simulink model "SensorlessBDC"  (R2025a)
settings: Solver=FixedStepDiscrete  StartTime=0.0  StopTime=1  RelTol=1e-3  EnableMultiTasking=on
undefined symbols (not defined in the file or in its folder): A, B, observer_params, pi_params, robot_params, tf_den, tf_num, Ts
libraries: simulink x4, mcbhdlcontrolslib x2, SignalEditorBlockLib x1
settings Model: Creator=Evan Wu  LastModifiedBy=Evan Wu
settings SolverCC: AutoInsertRateTranBlk=on
settings DataIOCC: SaveOutput=off  SaveTime=off
settings OptimizationCC: DefaultParameterBehavior=Inlined  InlineInvariantSignals=on  EnhancedBackFolding=on  PassReuseOutputArgsAs=Individual arguments  StateBitsets=on  DataBitsets=on  ZeroExternalMemoryAtStartup=off  ZeroInternalMemoryAtStartup=off  NoFixptDivByZeroProtection=on  LifeSpan=1  OptimizeBlockOrder=speed  DifferentSizesBufferReuse=on  EfficientTunableParamExpr=on
settings DebuggingCC: AlgebraicLoopMsg=error  ParameterTunabilityLossMsg=error
settings HardwareCC: ProdBitPerPointer=32.0  ProdBitPerSizeT=32.0  ProdBitPerPtrDiffT=32.0  ProdLargestAtomicFloat=None  ProdIntDivRoundTo=Floor  ProdWordSize=32.0  ProdHWDeviceType=Generic->Custom
settings SFSimCC: MATLABDynamicMemAlloc=off
settings RTWCC: SystemTargetFile=ert.tlc  TLCOptions=-p0  GenCodeOnly=on  TemplateMakefile=ert_default_tmf  GenerateReport=on  RTWVerbose=off  IncludeHyperlinkInReport=on  LaunchReport=on  Description=Embedded Coder
settings CodeAppCC: ForceParamTrailComments=on  IgnoreCustomStorageClasses=off  OperatorAnnotations=on  SimulinkDataObjDesc=on  SFDataObjDesc=on  CustomSymbolStrGlobalVar=rt$N$M  CustomSymbolStrType=$N$M  CustomSymbolStrFcn=$N$M$F  CustomSymbolStrMacro=$N$M  InsertBlockDesc=on
settings ERTTargetCC: ExtModeTransport=0.0  ExtModeStaticAlloc=off  ExtModeMexFile=ext_comm  ExtModeIntrfLevel=Level1  RootIOFormat=Structure reference  ERTCustomFileTemplate=example_file_process.tlc  TargetLangStandard=C99 (ISO)  CodeReplacementLibrary=ISO_C  GenerateSampleERTMain=on  IncludeMdlTerminateFcn=off  SuppressErrorStatus=on  SupportAbsoluteTime=off  PurelyIntegerCode=on  SupportNonFinite=off  SupportComplex=off

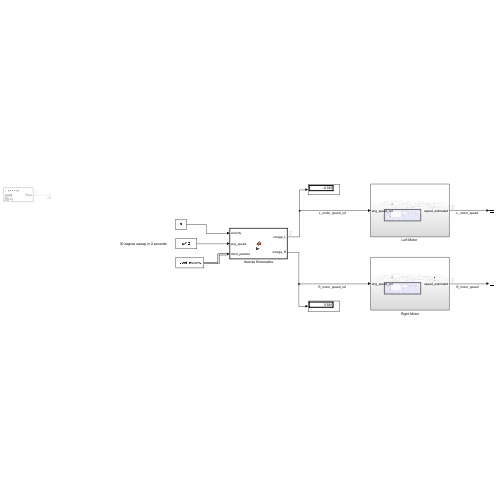
[thumbnail: Simulink's stored preview of the top-level diagram]
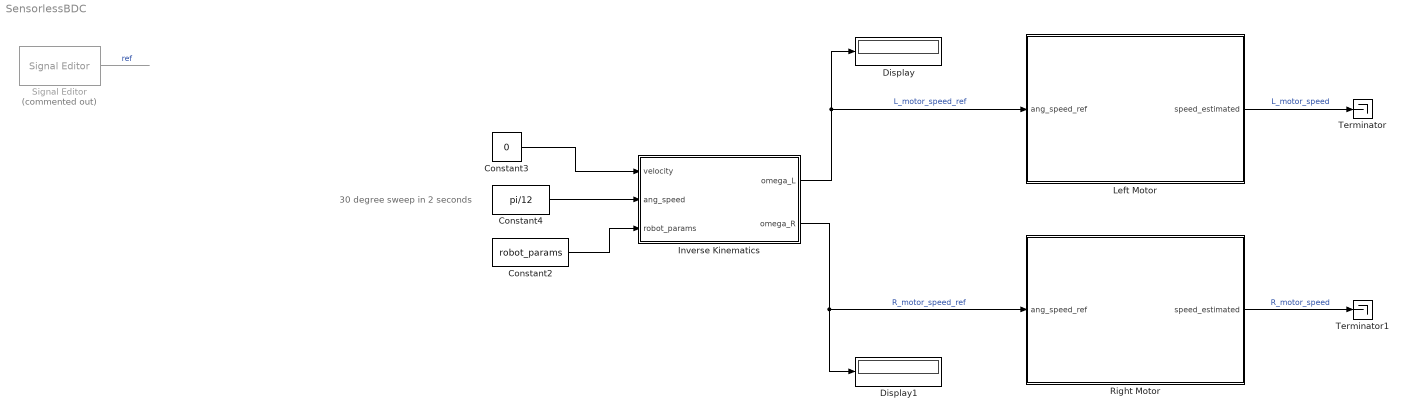
== system SensorlessBDC ==
  note: 30 degree sweep in 2 seconds
  Constant2 : Constant  Value=robot_params  OutDataTypeStr=Bus: slBus3
  Constant3 : Constant  Value=0
  Constant4 : Constant  Value=pi/12
  Display : Display
  Display1 : Display
  Inverse Kinematics : MATLAB Function  TreatAsAtomicUnit=on
  "Left Motor " : Subsystem
  Right Motor : Subsystem
  Signal Editor : SignalEditorBlockLib/Signal Editor  Commented=on  FileName=step_response.mat  ActiveScenario=Scenario  ActiveSignal=Step  IsBus=off  OutputBusObjectStr=Bus: BusObject  SampleTime=0  ZeroCross=off  OutputAfterFinalValue=Setting to zero  Unit=inherit  PreserveSignalName=on  ApplySigPropsToAllScenarios=on  ApplySigPropsToAllSignals=off  SignalPropertySource=Dialog parameters
  Terminator : Terminator
  Terminator1 : Terminator
  wires:
  Signal Editor/1 -> ?  "ref"
  Constant2/1 -> Inverse Kinematics/3(robot_params)
  Constant3/1 -> Inverse Kinematics/1(velocity)
  Constant4/1 -> Inverse Kinematics/2(ang_speed)
  Inverse Kinematics/2(omega_R) -> Display1/1, Right Motor/1(ang_speed_ref)  "R_motor_speed_ref"
  Inverse Kinematics/1(omega_L) -> "Left Motor "/1(ang_speed_ref), Display/1  "L_motor_speed_ref"
  "Left Motor "/1(speed_estimated) -> Terminator/1  "L_motor_speed"
  Right Motor/1(speed_estimated) -> Terminator1/1  "R_motor_speed"

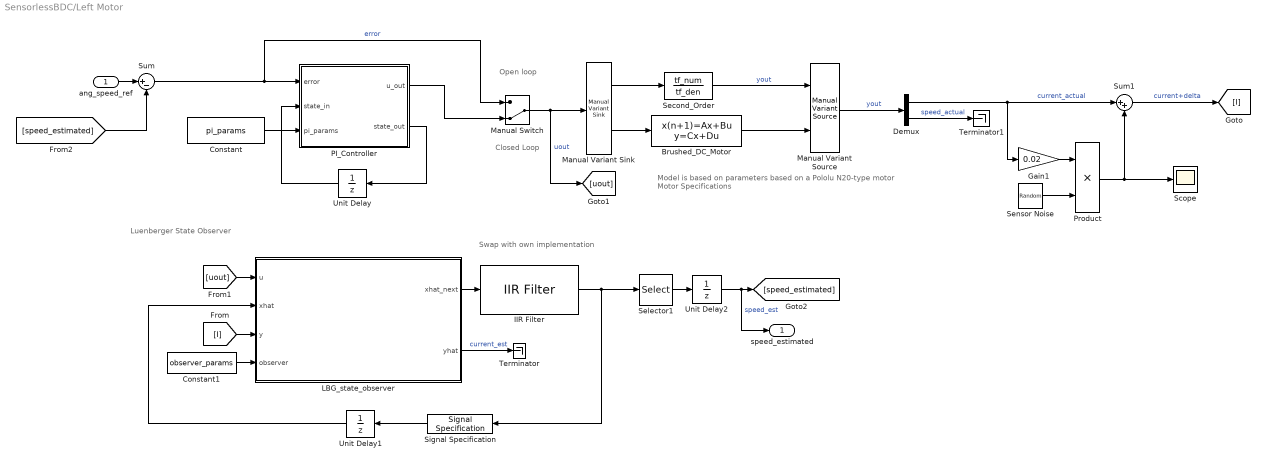
== system SensorlessBDC/Left Motor  ==
  note: Swap with own implementation
  note: Model is based on parameters based on a Pololu N20-type motor
      | Motor Specifications
  note: Luenberger State Observer
  note: Closed Loop
  note: Open loop
  ang_speed_ref : Inport
  Brushed_DC_Motor : DiscreteStateSpace  A=A  B=B  C=[1 0 ; 0 1]  D=zeros(2,1)  SampleTime=Ts/10
  Constant : Constant  Value=pi_params  VectorParams1D=off  OutDataTypeStr=Bus: slBus1  SampleTime=-1
  Constant1 : Constant  Value=observer_params  OutDataTypeStr=Bus: slBus2  SampleTime=-1
  Demux : Demux  Outputs=2
  Gain1 : Gain  Gain=0.02
  IIR Filter : mcbhdlcontrolslib/IIR Filter  VariantControl=Low Pass Filter  VariantSelect=Low-pass  FilterConstantInputType=Specify via dialog  Filter_constant=0.05  advancedSettings=on  Ts=Ts  cutOff_freq=80.4151
      settings: LibrarySourceBlock=mcbhdllib/Signal Management/IIR Filter
  LBG_state_observer : MATLAB Function  TreatAsAtomicUnit=on
  Manual Variant Sink : simulink/Signal Routing/Manual Variant Sink  NumChoices=2  LabelModeActiveChoice=V_2
  Manual Variant Source : simulink/Signal Routing/Manual Variant Source  NumChoices=2  LabelModeActiveChoice=V_2
  Manual Switch : ManualSwitch  CurrentSetting=0
  PI_Controller : MATLAB Function  TreatAsAtomicUnit=on
  Product : Product
  Scope : Scope
      settings: ActiveDisplayYMinimum=-0.5016078017590786  ActiveDisplayYMaximum=0.51010251517112981
  Second_Order : TransferFcn  Numerator=tf_num  Denominator=tf_den
  Selector1 : Selector  NumberOfDimensions=2  InputPortWidth=3  IndexOptions=Index vector (dialog),Index vector (dialog)  Indices=2,1  OutputSizes=1,1
  Sensor Noise : RandomNumber  Seed=42  SampleTime=Ts
  Signal Specification : SignalSpecification  Dimensions=[2 1]
  Sum : Sum  Inputs=|+-
  Sum1 : Sum  Inputs=|++
  Terminator : Terminator
  Terminator1 : Terminator
  Unit Delay : UnitDelay  SampleTime=-1  HasFrameUpgradeWarning=on
  Unit Delay1 : UnitDelay  SampleTime=-1  HasFrameUpgradeWarning=on
  Unit Delay2 : UnitDelay  SampleTime=-1  HasFrameUpgradeWarning=on
  speed_estimated : Outport
  wires:
  PI_Controller/2(state_out) -> Unit Delay/1
  Manual Variant Sink/1 -> Second_Order/1
  Product/1 -> Sum1/2, Scope/1
  Manual Switch/1 -> [uout], Manual Variant Sink/1  "uout"
  Constant1/1 -> LBG_state_observer/4(observer)
  Manual Variant Sink/2 -> Brushed_DC_Motor/1
  Demux/1 -> Sum1/1, Gain1/1  "current_actual"
  Unit Delay/1 -> PI_Controller/2(state_in)
  Unit Delay1/1 -> LBG_state_observer/2(xhat)
  [uout] -> LBG_state_observer/1(u)
  Sum1/1 -> [I]  "current+delta"
  Sum/1 -> Manual Switch/1, PI_Controller/1(error)  "error"
  Selector1/1 -> Unit Delay2/1
  Gain1/1 -> Product/1
  LBG_state_observer/2(yhat) -> Terminator/1  "current_est"
  Demux/2 -> Terminator1/1  "speed_actual"
  ang_speed_ref/1 -> Sum/1
  Constant/1 -> PI_Controller/3(pi_params)
  [speed_estimated] -> Sum/2
  Brushed_DC_Motor/1 -> Manual Variant Source/2
  Signal Specification/1 -> Unit Delay1/1
  Manual Variant Source/1 -> Demux/1  "yout"
  Unit Delay2/1 -> speed_estimated/1, [speed_estimated]  "speed_est"
  [I] -> LBG_state_observer/3(y)
  PI_Controller/1(u_out) -> Manual Switch/2
  LBG_state_observer/1(xhat_next) -> IIR Filter/1
  Sensor Noise/1 -> Product/2
  IIR Filter/1 -> Signal Specification/1, Selector1/1
  Second_Order/1 -> Manual Variant Source/1  "yout"

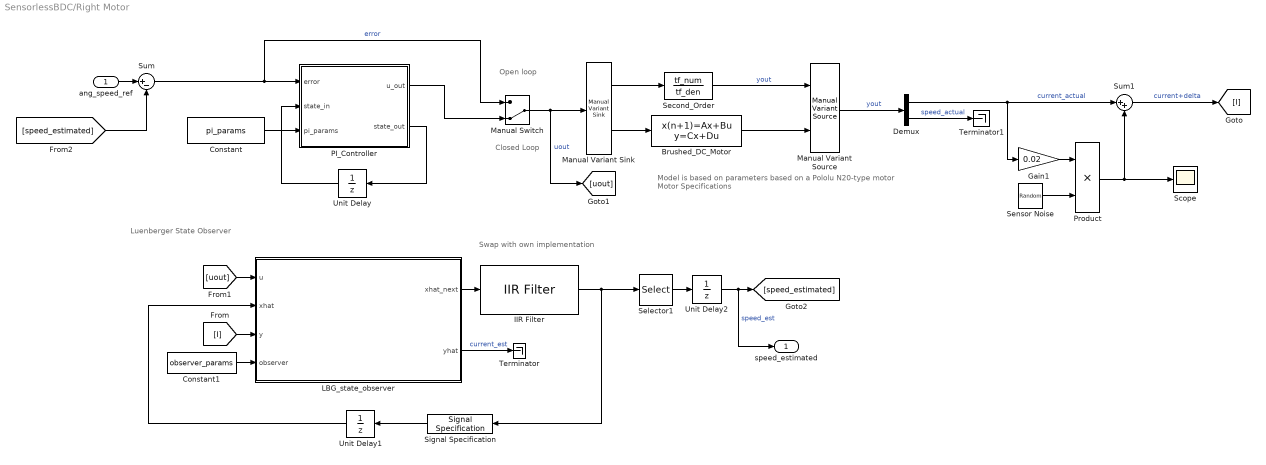
== system SensorlessBDC/Right Motor ==
  note: Swap with own implementation
  note: Model is based on parameters based on a Pololu N20-type motor
      | Motor Specifications
  note: Luenberger State Observer
  note: Closed Loop
  note: Open loop
  ang_speed_ref : Inport
  Brushed_DC_Motor : DiscreteStateSpace  A=A  B=B  C=[1 0 ; 0 1]  D=zeros(2,1)  SampleTime=Ts/10
  Constant : Constant  Value=pi_params  VectorParams1D=off  OutDataTypeStr=Bus: slBus1  SampleTime=-1
  Constant1 : Constant  Value=observer_params  OutDataTypeStr=Bus: slBus2  SampleTime=-1
  Demux : Demux  Outputs=2
  Gain1 : Gain  Gain=0.02
  IIR Filter : mcbhdlcontrolslib/IIR Filter  VariantControl=Low Pass Filter  VariantSelect=Low-pass  FilterConstantInputType=Specify via dialog  Filter_constant=0.05  advancedSettings=on  Ts=Ts  cutOff_freq=80.4151
      settings: LibrarySourceBlock=mcbhdllib/Signal Management/IIR Filter
  LBG_state_observer : MATLAB Function  TreatAsAtomicUnit=on
  Manual Variant Sink : simulink/Signal Routing/Manual Variant Sink  NumChoices=2  LabelModeActiveChoice=V_2
  Manual Variant Source : simulink/Signal Routing/Manual Variant Source  NumChoices=2  LabelModeActiveChoice=V_2
  Manual Switch : ManualSwitch  CurrentSetting=0
  PI_Controller : MATLAB Function  TreatAsAtomicUnit=on
  Product : Product
  Scope : Scope
      settings: ActiveDisplayYMinimum=-0.5016078017590786  ActiveDisplayYMaximum=0.51010251517112981
  Second_Order : TransferFcn  Numerator=tf_num  Denominator=tf_den
  Selector1 : Selector  NumberOfDimensions=2  InputPortWidth=3  IndexOptions=Index vector (dialog),Index vector (dialog)  Indices=2,1  OutputSizes=1,1
  Sensor Noise : RandomNumber  Seed=42  SampleTime=Ts
  Signal Specification : SignalSpecification  Dimensions=[2 1]
  Sum : Sum  Inputs=|+-
  Sum1 : Sum  Inputs=|++
  Terminator : Terminator
  Terminator1 : Terminator
  Unit Delay : UnitDelay  SampleTime=-1  HasFrameUpgradeWarning=on
  Unit Delay1 : UnitDelay  SampleTime=-1  HasFrameUpgradeWarning=on
  Unit Delay2 : UnitDelay  SampleTime=-1  HasFrameUpgradeWarning=on
  speed_estimated : Outport
  wires:
  PI_Controller/2(state_out) -> Unit Delay/1
  Manual Variant Sink/1 -> Second_Order/1
  Product/1 -> Sum1/2, Scope/1
  Manual Switch/1 -> [uout], Manual Variant Sink/1  "uout"
  Constant1/1 -> LBG_state_observer/4(observer)
  Manual Variant Sink/2 -> Brushed_DC_Motor/1
  Demux/1 -> Sum1/1, Gain1/1  "current_actual"
  Unit Delay/1 -> PI_Controller/2(state_in)
  Unit Delay1/1 -> LBG_state_observer/2(xhat)
  [uout] -> LBG_state_observer/1(u)
  Sum1/1 -> [I]  "current+delta"
  Sum/1 -> Manual Switch/1, PI_Controller/1(error)  "error"
  Selector1/1 -> Unit Delay2/1
  Gain1/1 -> Product/1
  LBG_state_observer/2(yhat) -> Terminator/1  "current_est"
  Demux/2 -> Terminator1/1  "speed_actual"
  ang_speed_ref/1 -> Sum/1
  Constant/1 -> PI_Controller/3(pi_params)
  [speed_estimated] -> Sum/2
  Brushed_DC_Motor/1 -> Manual Variant Source/2
  Signal Specification/1 -> Unit Delay1/1
  Manual Variant Source/1 -> Demux/1  "yout"
  Unit Delay2/1 -> speed_estimated/1, [speed_estimated]  "speed_est"
  [I] -> LBG_state_observer/3(y)
  PI_Controller/1(u_out) -> Manual Switch/2
  LBG_state_observer/1(xhat_next) -> IIR Filter/1
  Sensor Noise/1 -> Product/2
  IIR Filter/1 -> Signal Specification/1, Selector1/1
  Second_Order/1 -> Manual Variant Source/1  "yout"

== matlab function SensorlessBDC/Left Motor /LBG_state_observer ==
  data: xhat_next output; u input; xhat input size=[2 1]; y input; observer input Bus: slBus2; yhat output
function [xhat_next, yhat] = fcn(u, xhat, y, observer)

xhat_next = zeros(2,1);
yhat      = zeros(1,1);

[xhat_next, yhat] = lbg_state_observer(u,xhat, y, observer);
end

== matlab function SensorlessBDC/Left Motor /PI_Controller ==
  data: error input size=1; u_out output; state_in input size=1; state_out output size=1; pi_params input Bus: slBus1 size=1
function [u_out, state_out] = fcn(error, state_in, pi_params)

u_out = zeros(1,1);
state_out = zeros(1,1);

[u_out, state_out] = pi_controller(error, state_in, pi_params);
end

== matlab function SensorlessBDC/Inverse Kinematics ==
  data: velocity input; omega_L output; ang_speed input; robot_params input; omega_R output
function [omega_L, omega_R] = fcn(velocity, ang_speed, robot_params)
[omega_L, omega_R] = compute_wheel_speed(velocity, ang_speed, robot_params);
end

== matlab function SensorlessBDC/Right Motor/LBG_state_observer ==
  data: xhat_next output; u input; xhat input size=[2 1]; y input; observer input Bus: slBus2; yhat output
function [xhat_next, yhat] = fcn(u, xhat, y, observer)

xhat_next = zeros(2,1);
yhat      = zeros(1,1);

[xhat_next, yhat] = lbg_state_observer(u,xhat, y, observer);
end

== matlab function SensorlessBDC/Right Motor/PI_Controller ==
  data: error input size=1; u_out output; state_in input size=1; state_out output size=1; pi_params input Bus: slBus1 size=1
function [u_out, state_out] = fcn(error, state_in, pi_params)

u_out = zeros(1,1);
state_out = zeros(1,1);

[u_out, state_out] = pi_controller(error, state_in, pi_params);
end
